simulink model "sampleModel1971_2_sub_sub_sub"  (R2023a)
settings: Solver=VariableStepAuto  StartTime=0.0  StopTime=10.0  RelTol=1e-3
libraries: hdlsllib x6, simulink x1
settings Model: Creator=user1  LastModifiedBy=user1

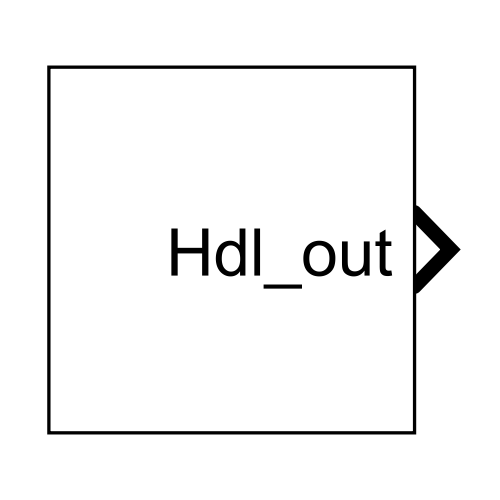
[thumbnail: Simulink's stored preview of the top-level diagram]
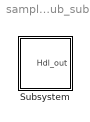
== system sampleModel1971_2_sub_sub_sub ==
  Subsystem : Subsystem

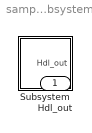
== system sampleModel1971_2_sub_sub_sub/Subsystem ==
  Subsystem : Subsystem
  Hdl_out : Outport  OutDataTypeStr=uint8

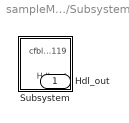
== system sampleModel1971_2_sub_sub_sub/Subsystem/Subsystem ==
  Subsystem : Subsystem
  Hdl_out : Outport  OutDataTypeStr=uint8

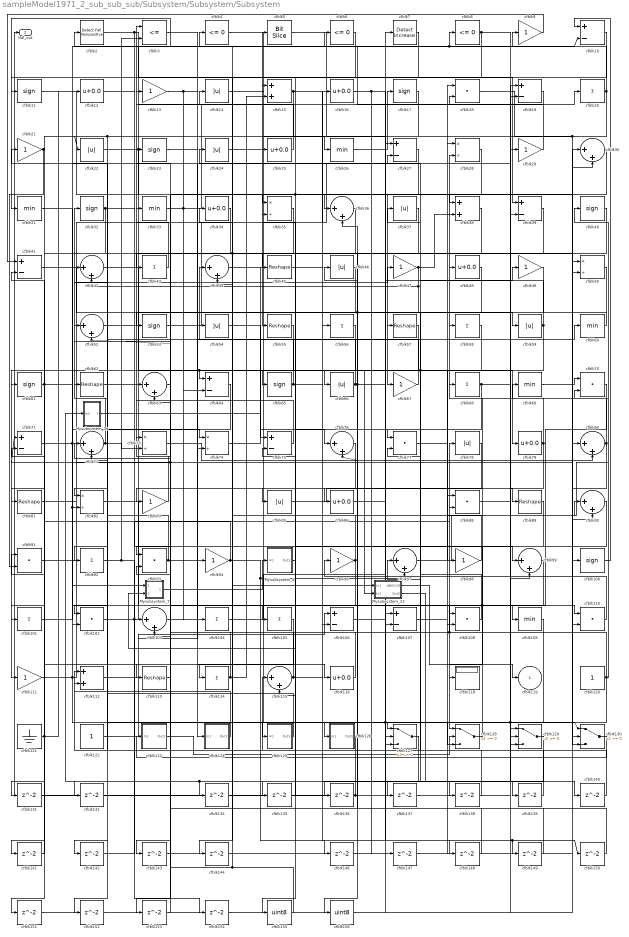
== system sampleModel1971_2_sub_sub_sub/Subsystem/Subsystem/Subsystem ==
  Mysubsystem_23 : Subsystem  TreatAsAtomicUnit=on  RTWFcnName=Mysubsystem_23
      settings: RTWFcnNameOpts=User specified  RTWFileNameOpts=Use function name
  Mysubsystem_39 : Subsystem  TreatAsAtomicUnit=on  RTWFcnName=Mysubsystem_39
      settings: RTWFcnNameOpts=User specified  RTWFileNameOpts=Use function name
  Mysubsystem_7 : Subsystem  TreatAsAtomicUnit=on  RTWFcnName=Mysubsystem_7
      settings: RTWFcnNameOpts=User specified  RTWFileNameOpts=Use function name
  Mysubsystem_8 : Subsystem  TreatAsAtomicUnit=on  RTWFcnName=Mysubsystem_8
      settings: RTWFcnNameOpts=User specified  RTWFileNameOpts=Use function name
  cfblk{10,19,27,39,41,64,71,75,106..107} (10 alike) : Sum  Inputs=+-  OutDataTypeStr=uint8
  cfblk{11,17,23,32,40,53,61,65,100} (9 alike) : Signum
  cfblk{20,43,56,58,68,92,101,104..105,114} (10 alike) : Sum  Inputs=+  OutDataTypeStr=uint8
  cfblk{18,70,77,88,91,93,102,108,110} (9 alike) : DotProduct  OutDataTypeStr=uint8
  cfblk{30,36,42,44,52,63,72,76,80,90,97,99,103,115} (14 alike) : Sum  Inputs=|++  OutDataTypeStr=uint8
  cfblk{26,31,33,60,69,109} (6 alike) : MinMax  OutDataTypeStr=uint8
  cfblk{9,13,21,29,47,49,67,83,94,96,98,111} (12 alike) : Gain  OutDataTypeStr=uint8
  cfblk112 : Sum  OutDataTypeStr=uint8
  cfblk{45,55,57,62,81,89,113} (7 alike) : Reshape
  cfblk{12,16,25,34,48,79,86,116} (8 alike) : Bias  Bias=0.0  SaturateOnIntegerOverflow=off
  cfblk118 : Display
  cfblk120 : Constant  OutDataTypeStr=uint8  SampleTime=-1
  cfblk121 : Ground
  cfblk122 : Constant  OutDataTypeStr=uint8  SampleTime=-1
  cfblk123 : Subsystem
      settings: LibrarySourceBlock=|
      | hdlsllib/Ports &
      | Subsystems/Subsystem
  cfblk124 : Subsystem
      settings: LibrarySourceBlock=|
      | hdlsllib/Ports &
      | Subsystems/Subsystem
  cfblk125 : Subsystem
      settings: LibrarySourceBlock=|
      | hdlsllib/Ports &
      | Subsystems/Subsystem
  cfblk126 : Subsystem
      settings: LibrarySourceBlock=|
      | hdlsllib/Ports &
      | Subsystems/Subsystem
  cfblk{127..130} (4 alike) : Switch  OutDataTypeStr=uint8  SaturateOnIntegerOverflow=off  InputSameDT=off
  cfblk{131..132,134..144,146..154} (22 alike) : Delay  SampleTime=1
  cfblk{14,22,24,37,46,54,59,66,78,85} (10 alike) : Abs  OutDataTypeStr=uint8  SaturateOnIntegerOverflow=off
  cfblk15 : Sum  OutDataTypeStr=uint8
  cfblk155 : DataTypeConversion  OutDataTypeStr=uint8  SaturateOnIntegerOverflow=off  RndMeth=Floor
  cfblk156 : DataTypeConversion  OutDataTypeStr=uint8  SaturateOnIntegerOverflow=off  RndMeth=Floor
  cfblk2 : hdlsllib/Logic and Bit Operations/Detect Fall Nonpositive  vinit=0  OutDataTypeStr=uint8
  cfblk{28,35,50,73..74,82} (6 alike) : Product  Inputs=*/  OutDataTypeStr=uint8  RndMeth=Zero  SaturateOnIntegerOverflow=on
  cfblk3 : RelationalOperator  Operator=<=  OutDataTypeStr=boolean  InputSameDT=off
  cfblk38 : Sum  OutDataTypeStr=uint8
  cfblk4 : hdlsllib/Logic and Bit Operations/Compare To Zero  relop=<=  OutDataTypeStr=uint8
  cfblk5 : hdlsllib/Logic and Bit Operations/Bit Slice  lidx=7  ridx=0
  cfblk6 : hdlsllib/Logic and Bit Operations/Compare To Zero  relop=<=  OutDataTypeStr=uint8
  cfblk7 : simulink/Logic and Bit Operations/Detect Increase  vinit=0.0  OutDataTypeStr=uint8
      settings: LibrarySourceBlock=|
      | hdlsllib/Logic and Bit
      | Operations/Detect
      | Increase
  cfblk8 : hdlsllib/Logic and Bit Operations/Compare To Zero  relop=<=  OutDataTypeStr=uint8
  cfblk119 : Outport  OutDataTypeStr=uint8  VectorParamsAs1DForOutWhenUnconnected=off
  Hdl_out : Outport  Port=2  OutDataTypeStr=uint8
  wires:
  cfblk13/1 -> cfblk127/2, cfblk104/1
  cfblk41/1 -> cfblk59/1
  cfblk14/1 -> cfblk126/1(In1)
  cfblk92/1 -> cfblk154/1, cfblk3/2
  cfblk2/1 -> cfblk50/2, cfblk39/1
  cfblk20/1 -> cfblk31/1, cfblk130/2, cfblk74/2
  cfblk4/1 -> cfblk26/1
  cfblk102/1 -> cfblk88/2, cfblk14/1
  cfblk28/1 -> cfblk67/1
  cfblk83/1 -> cfblk3/1
  cfblk3/1 -> cfblk124/1(In1)
  cfblk44/1 -> cfblk5/1
  cfblk88/1 -> cfblk29/1
  cfblk58/1 -> cfblk137/1, Mysubsystem_23/2(In2)
  cfblk62/1 -> cfblk15/1
  cfblk65/1 -> cfblk127/3, cfblk21/1
  cfblk97/1 -> cfblk40/1
  cfblk81/1 -> cfblk47/1
  cfblk103/1 -> cfblk60/1
  cfblk33/1 -> cfblk64/2, cfblk20/1
  cfblk108/1 -> cfblk24/1
  cfblk85/1 -> cfblk89/1
  cfblk24/1 -> cfblk66/1
  cfblk73/1 -> cfblk80/2
  cfblk43/1 -> cfblk33/1
  cfblk39/1 -> cfblk55/1
  cfblk72/1 -> cfblk73/2, cfblk32/1
  cfblk55/1 -> cfblk111/1
  cfblk74/1 -> cfblk45/1
  cfblk8/1 -> cfblk11/1, cfblk140/1, cfblk130/1
  cfblk35/1 -> cfblk141/1, Mysubsystem_23/1(In1)
  cfblk15/1 -> cfblk56/1, cfblk92/1, cfblk22/1
  cfblk26/1 -> cfblk17/1
  cfblk122/1 -> cfblk106/1
  cfblk126/1(Out1) -> cfblk115/1
  cfblk10/1 -> cfblk35/1
  cfblk46/1 -> cfblk65/1
  cfblk113/1 -> cfblk73/1
  cfblk70/1 -> cfblk109/1
  cfblk99/1 -> cfblk118/1, cfblk103/2
  cfblk111/1 -> cfblk130/3, cfblk19/1
  cfblk104/1 -> cfblk49/1
  cfblk75/1 -> cfblk63/1
  cfblk120/1 -> cfblk127/1, cfblk70/2, cfblk52/1, cfblk78/1
  cfblk37/1 -> cfblk86/1
  cfblk42/1 -> cfblk88/1
  cfblk11/1 -> cfblk106/2
  cfblk112/1 -> cfblk94/1
  cfblk114/1 -> cfblk15/2, cfblk72/1
  cfblk124/1(Out1) -> cfblk112/1
  cfblk9/1 -> cfblk41/1
  cfblk89/1 -> cfblk105/1
  cfblk121/1 -> cfblk12/1, cfblk91/1
  cfblk40/1 -> cfblk81/1
  cfblk82/1 -> cfblk128/1
  cfblk21/1 -> cfblk91/2, cfblk61/1
  cfblk22/1 -> cfblk100/1, cfblk9/1
  cfblk96/1 -> cfblk125/1(In1), cfblk13/1
  cfblk52/1 -> cfblk79/1
  cfblk7/1 -> cfblk155/1
  cfblk116/1 -> cfblk35/2
  cfblk110/1 -> cfblk96/1
  cfblk59/1 -> cfblk37/1, cfblk82/1, cfblk64/1
  cfblk54/1 -> cfblk76/1
  cfblk77/1 -> cfblk98/1
  cfblk80/1 -> cfblk110/2, cfblk28/2
  cfblk50/1 -> cfblk53/1
  cfblk128/1 -> cfblk68/1
  cfblk17/1 -> cfblk101/1
  cfblk56/1 -> cfblk102/1
  cfblk38/1 -> cfblk82/2, Mysubsystem_7/1(In1)
  cfblk30/1 -> cfblk83/1, cfblk85/1
  cfblk129/1 -> cfblk134/1, Mysubsystem_39/1(In1)
  cfblk5/1 -> cfblk107/2
  cfblk93/1 -> cfblk42/1, cfblk27/2
  cfblk27/1 -> cfblk36/1
  cfblk57/1 -> cfblk113/1
  cfblk48/1 -> cfblk77/1
  cfblk79/1 -> cfblk129/3, cfblk69/1
  cfblk16/1 -> cfblk147/1, cfblk148/1, cfblk129/2
  cfblk86/1 -> cfblk58/1
  cfblk19/1 -> cfblk18/2
  cfblk36/1 -> cfblk114/1
  cfblk53/1 -> cfblk16/1
  cfblk12/1 -> cfblk38/1
  cfblk68/1 -> cfblk135/1, cfblk129/1
  cfblk66/1 -> cfblk54/1, cfblk46/1, cfblk48/1
  cfblk32/1 -> cfblk102/2, cfblk99/1
  cfblk115/1 -> cfblk138/1, cfblk52/2, cfblk71/1
  cfblk71/1 -> cfblk128/3, cfblk25/1
  cfblk90/1 -> cfblk108/1
  cfblk107/1 -> cfblk90/1
  cfblk125/1(Out1) -> cfblk62/1
  cfblk123/1(Out1) -> cfblk128/2
  cfblk23/1 -> cfblk116/1
  cfblk31/1 -> cfblk110/1
  cfblk100/1 -> cfblk10/1
  cfblk67/1 -> cfblk44/1
  cfblk94/1 -> cfblk41/2, cfblk146/1, cfblk97/2
  cfblk25/1 -> cfblk4/1
  cfblk34/1 -> cfblk43/1
  cfblk29/1 -> cfblk6/1
  cfblk45/1 -> cfblk150/1, cfblk149/1
  cfblk101/1 -> cfblk10/2, cfblk8/1
  cfblk47/1 -> cfblk38/2, cfblk42/2, cfblk76/2, cfblk115/2
  cfblk130/1 -> cfblk123/1(In1)
  cfblk60/1 -> cfblk57/1
  cfblk91/1 -> cfblk30/1
  cfblk61/1 -> cfblk151/1, cfblk74/1
  cfblk69/1 -> cfblk70/1
  cfblk98/1 -> cfblk2/1
  cfblk18/1 -> cfblk30/2
  cfblk63/1 -> cfblk93/1
  cfblk105/1 -> cfblk131/1
  cfblk131/1 -> cfblk27/1
  cfblk64/1 -> cfblk132/1
  cfblk132/1 -> cfblk28/1
  cfblk134/1 -> cfblk108/2
  cfblk135/1 -> cfblk75/2
  cfblk136/1 -> Hdl_out/1, cfblk72/2
  cfblk137/1 -> cfblk19/2
  cfblk138/1 -> cfblk77/2
  cfblk106/1 -> cfblk139/1
  cfblk139/1 -> cfblk97/1
  cfblk140/1 -> cfblk112/2
  cfblk141/1 -> cfblk71/2
  cfblk109/1 -> cfblk142/1
  cfblk142/1 -> cfblk103/1
  cfblk76/1 -> cfblk143/1
  cfblk143/1 -> cfblk18/1
  cfblk6/1 -> cfblk144/1
  cfblk144/1 -> cfblk39/2
  cfblk146/1 -> cfblk90/2
  cfblk147/1 -> cfblk50/1
  cfblk148/1 -> cfblk93/2
  cfblk149/1 -> cfblk44/2
  cfblk150/1 -> cfblk36/2
  cfblk151/1 -> cfblk99/2
  cfblk127/1 -> cfblk152/1
  cfblk152/1 -> cfblk107/1
  cfblk49/1 -> cfblk153/1
  cfblk153/1 -> cfblk63/2
  cfblk154/1 -> cfblk80/1
  cfblk155/1 -> cfblk34/1, cfblk23/1
  cfblk78/1 -> cfblk156/1
  cfblk156/1 -> cfblk7/1
  Mysubsystem_7/1(Out1) -> Mysubsystem_8/1(In1)
  Mysubsystem_8/1(Out1) -> Mysubsystem_7/2(In2)
  Mysubsystem_23/1(cfblk119) -> cfblk119/1
  Mysubsystem_23/2(Out2) -> cfblk136/1
  Mysubsystem_39/1(Y) -> cfblk75/1

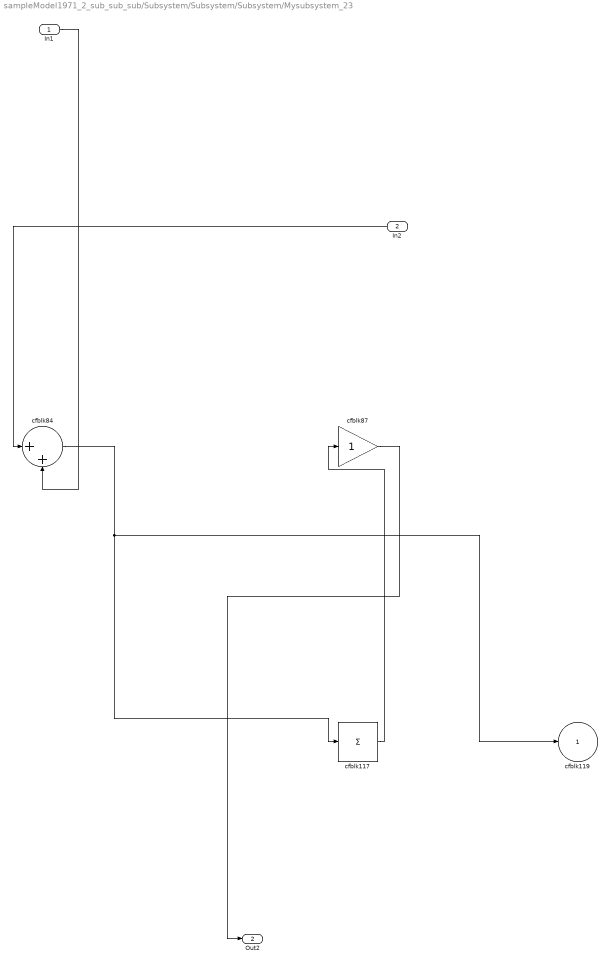
== system sampleModel1971_2_sub_sub_sub/Subsystem/Subsystem/Subsystem/Mysubsystem_23 ==
  In1 : Inport
  In2 : Inport  Port=2
  cfblk117 : Sum  Inputs=+
  cfblk84 : Sum  Inputs=|++
  cfblk87 : Gain
  cfblk119 : Outport  VectorParamsAs1DForOutWhenUnconnected=off
  Out2 : Outport  Port=2
  wires:
  In2/1 -> cfblk84/1
  cfblk117/1 -> cfblk87/1
  In1/1 -> cfblk84/2
  cfblk87/1 -> Out2/1
  cfblk84/1 -> cfblk117/1, cfblk119/1

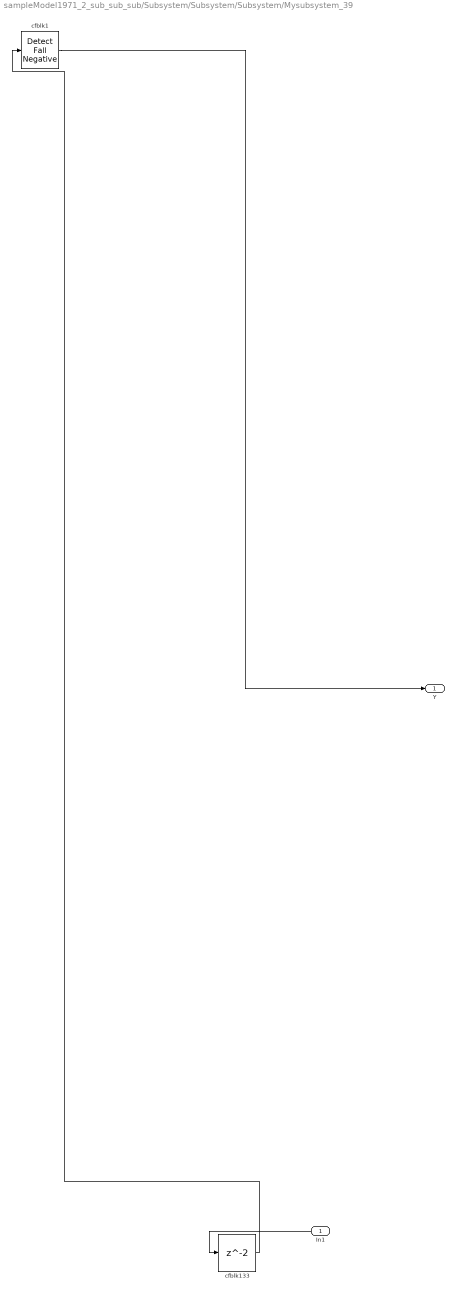
== system sampleModel1971_2_sub_sub_sub/Subsystem/Subsystem/Subsystem/Mysubsystem_39 ==
  In1 : Inport
  cfblk1 : hdlsllib/Logic and Bit Operations/Detect Fall Negative  vinit=0  OutDataTypeStr=boolean
  cfblk133 : Delay  SampleTime=1
  Y : Outport
  wires:
  In1/1 -> cfblk133/1
  cfblk1/1 -> Y/1
  cfblk133/1 -> cfblk1/1

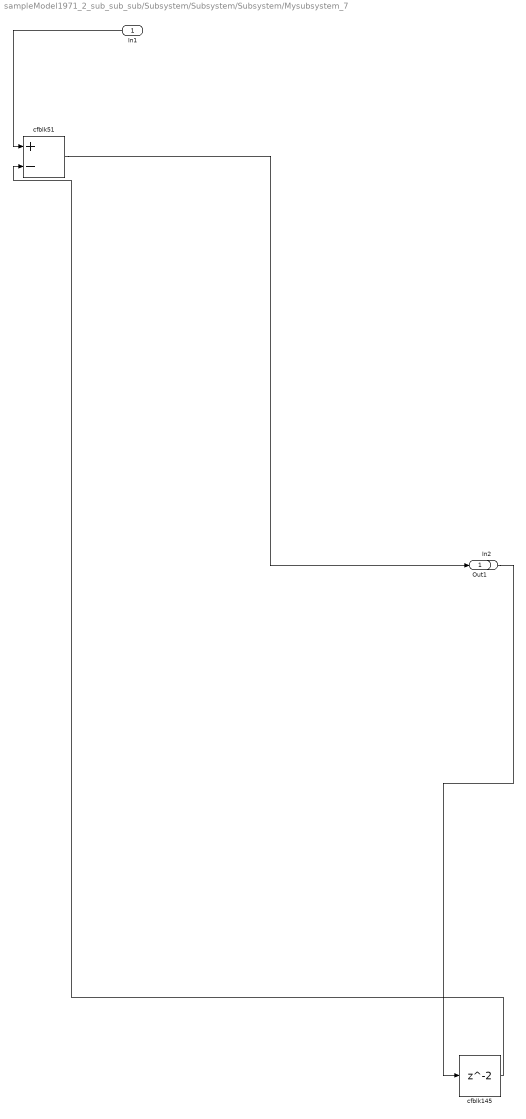
== system sampleModel1971_2_sub_sub_sub/Subsystem/Subsystem/Subsystem/Mysubsystem_7 ==
  In1 : Inport
  In2 : Inport  Port=2
  cfblk145 : Delay  SampleTime=1
  cfblk51 : Sum  Inputs=+-
  Out1 : Outport
  wires:
  cfblk51/1 -> Out1/1
  In2/1 -> cfblk145/1
  In1/1 -> cfblk51/1
  cfblk145/1 -> cfblk51/2

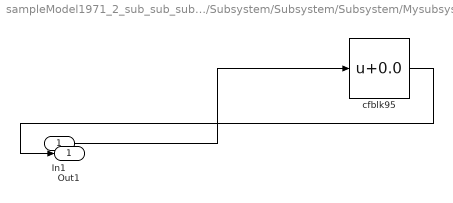
== system sampleModel1971_2_sub_sub_sub/Subsystem/Subsystem/Subsystem/Mysubsystem_8 ==
  In1 : Inport
  cfblk95 : Bias  Bias=0.0  SaturateOnIntegerOverflow=off
  Out1 : Outport
  wires:
  In1/1 -> cfblk95/1
  cfblk95/1 -> Out1/1

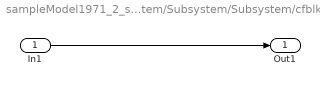
== system sampleModel1971_2_sub_sub_sub/Subsystem/Subsystem/Subsystem/cfblk123 ==
  In1 : Inport
  Out1 : Outport
  wires:
  In1/1 -> Out1/1

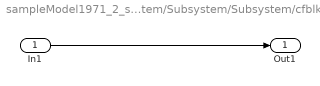
== system sampleModel1971_2_sub_sub_sub/Subsystem/Subsystem/Subsystem/cfblk124 ==
  In1 : Inport
  Out1 : Outport
  wires:
  In1/1 -> Out1/1

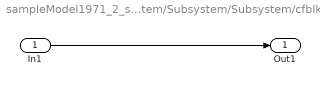
== system sampleModel1971_2_sub_sub_sub/Subsystem/Subsystem/Subsystem/cfblk125 ==
  In1 : Inport
  Out1 : Outport
  wires:
  In1/1 -> Out1/1

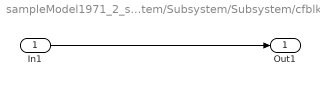
== system sampleModel1971_2_sub_sub_sub/Subsystem/Subsystem/Subsystem/cfblk126 ==
  In1 : Inport
  Out1 : Outport
  wires:
  In1/1 -> Out1/1
